simulink model "coil_ironcore_b"  (R2024a)
settings: Solver=VariableStepAuto  StartTime=0.0  StopTime=te  MaxStep=te/500  RelTol=1e-3
values from neighbouring files (symbols this model uses):
  A = 9e-4    (= 0.0009)    [Electromagnet_par.m]    (also in coil_ironcore.m = 0.0005; sim21_ODE.m = 2)
  B = [0.062749, 0.13454, 0.28376, 0.56098, 0.93453, 1.2404, 1.413, 1.497,1.5364, 1.5549]    [Electromagnet_par.m]    (also in coil_ironcore.m = [-fliplr(B) 0 B])
  H = [10, 21.544, 46.416, 100, 215.44, 464.16, 1000, 2154.4, 4641.6, 10000]    [Electromagnet_par.m]    (also in coil_ironcore.m = [-fliplr(H) 0 H])
  l = 2*pi*0.1    (= 0.628318530718)    [coil_ironcore.m]
  N = 900    [Electromagnet_par.m]    (also in coil_ironcore.m = 1000)
  R = 6.5    [Electromagnet_par.m]    (also in coil_ironcore.m = 10; sim21_ODE.m = 10)
  U = 10    [Electromagnet_par.m]    (also in coil_ironcore.m = 163; sim21_ODE.m = 230*sqrt(2))
  w = 2*pi/0.1    (= 62.8318530718)    [Electromagnet_par.m]    (also in coil_ironcore.m = 314.159265359; sim21_ODE.m = [0.5 1 2])
settings Model: Creator=ocean  LastModifiedBy=ocean

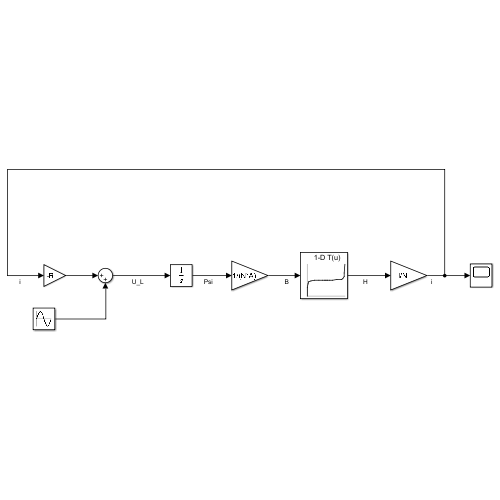
[thumbnail: Simulink's stored preview of the top-level diagram]
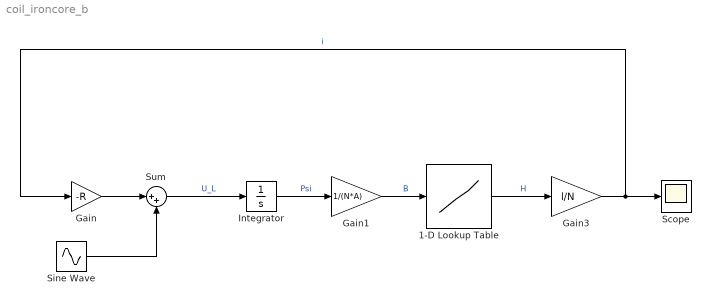
== system coil_ironcore_b ==
  1-D Lookup Table : Lookup_n-D  NumberOfTableDimensions=1  BreakpointsForDimension1=B  Table=H  InternalRulePriority=Speed  RndMeth=Simplest
  Gain : Gain  Gain=-R
  Gain1 : Gain  Gain=1/(N*A)
  Gain3 : Gain  Gain=l/N
  Integrator : Integrator
  Scope : Scope
  Sine Wave : Sin  Amplitude=U  Frequency=w  SampleTime=0
  Sum : Sum  Inputs=|++
  wires:
  Sine Wave/1 -> Sum/2
  Gain/1 -> Sum/1
  Sum/1 -> Integrator/1  "U_L"
  Integrator/1 -> Gain1/1  "Psi"
  Gain1/1 -> 1-D Lookup Table/1  "B"
  1-D Lookup Table/1 -> Gain3/1  "H"
  Gain3/1 -> Gain/1, Scope/1  "i"
